simulink model "spring_mass_damper_system"  (R2022a)
settings: Solver=VariableStepAuto  StartTime=0.0  StopTime=120  MaxStep=0.001  RelTol=1e-3
settings Model: Creator=alexandroslioulemes  LastModifiedBy=alexandroslioulemes

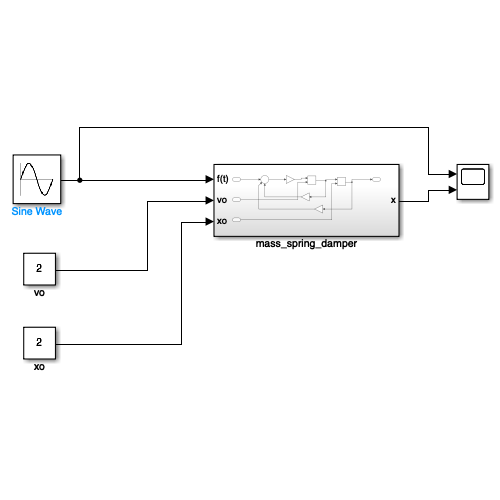
[thumbnail: Simulink's stored preview of the top-level diagram]
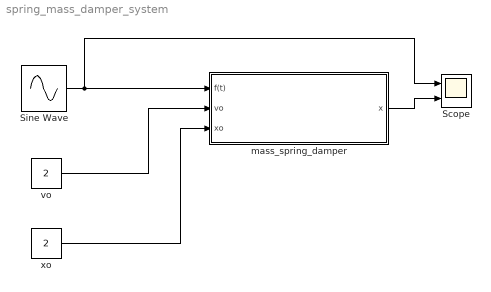
== system spring_mass_damper_system ==
  Scope : Scope  NumInputPorts=2
  Sine Wave : Sin  Amplitude=2  SampleTime=0
  mass_spring_damper : Subsystem
  vo : Constant  Value=2
  xo : Constant  Value=2
  wires:
  Sine Wave/1 -> mass_spring_damper/1(f(t)), Scope/1
  vo/1 -> mass_spring_damper/2(vo)
  xo/1 -> mass_spring_damper/3(xo)
  mass_spring_damper/1(x) -> Scope/2

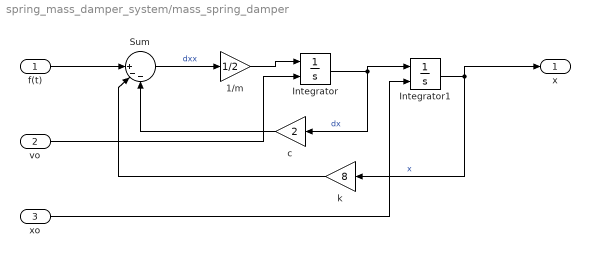
== system spring_mass_damper_system/mass_spring_damper ==
  f(t) : Inport
  vo : Inport  Port=2
  xo : Inport  Port=3
  1/m : Gain  Gain=1/2
  Integrator : Integrator  InitialConditionSource=external  InitialCondition=2
  Integrator1 : Integrator  InitialConditionSource=external  InitialCondition=1
  Sum : Sum  Inputs=||+--
  c : Gain  Gain=2
  k : Gain  Gain=8
  x : Outport
  wires:
  f(t)/1 -> Sum/1
  xo/1 -> Integrator1/2
  Integrator1/1 -> x/1, k/1  "x"
  vo/1 -> Integrator/2
  Sum/1 -> 1/m/1  "dxx"
  k/1 -> Sum/2
  1/m/1 -> Integrator/1
  c/1 -> Sum/3
  Integrator/1 -> Integrator1/1, c/1  "dx"
